simulink model "Problem_4"  (R2020a)
settings: Solver=ode45  StartTime=0.0  StopTime=0.2  RelTol=1e-3
PreLoadFcn:
  | J = 3.2284E-6;
  | b = 3.5077E-6;
  | K = 0.0274;
  | R = 4;
  | L = 2.75E-6;
  | Kp=4.02355957969103;
  | Ki=62.7263213782013;
  | Kd=0.0508488040948506;
settings Model: Creator=Ganesh  LastModifiedBy=Ganesh

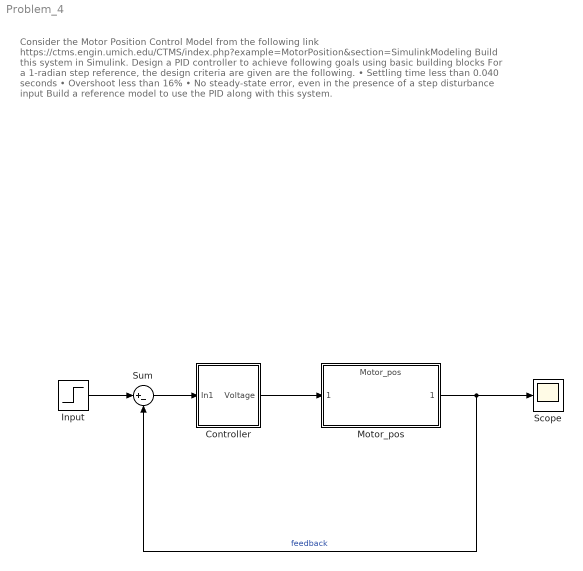
== system Problem_4 ==
  note: Consider the Motor Position Control Model from the following link https://ctms.engin.umich.edu/CTMS/index.php?example=MotorPosition&section=SimulinkModeling Build this system in Simulink.
      | Design a PID controller to achieve following goals using basic building blocks
      | For a 1-radian step reference, the design criteria are given are the following.
      | • Settling time less than 0.040 seconds
      | • Overshoot less than 16%
      | • No steady-state error, even in the presence of a step disturbance input
      | Build a reference model to use the PID along with this system.
  Controller : Subsystem
  Input : Step  Time=0  SampleTime=0
  Motor_pos : ModelReference  ModelNameDialog=Motor_pos  ModelReferenceVersion=1.8
  Scope : Scope
  Sum : Sum  Inputs=|+-
  wires:
  Motor_pos/1 -> Sum/2, Scope/1  "feedback"
  Input/1 -> Sum/1
  Sum/1 -> Controller/1(In1)
  Controller/1(Voltage) -> Motor_pos/1

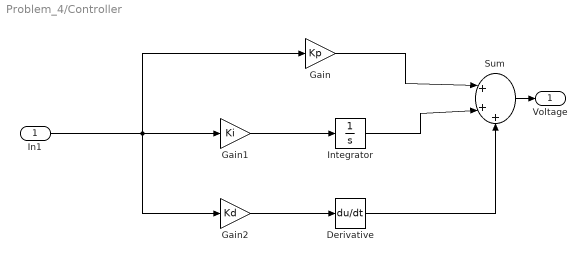
== system Problem_4/Controller ==
  In1 : Inport
  Derivative : Derivative
  Gain : Gain  Gain=Kp
  Gain1 : Gain  Gain=Ki
  Gain2 : Gain  Gain=Kd
  Integrator : Integrator
  Sum : Sum  Inputs=|+++
  Voltage : Outport
  wires:
  Gain/1 -> Sum/1
  In1/1 -> Gain2/1, Gain1/1, Gain/1
  Sum/1 -> Voltage/1
  Gain1/1 -> Integrator/1
  Gain2/1 -> Derivative/1
  Integrator/1 -> Sum/2
  Derivative/1 -> Sum/3
